simulink model "BLOC_Platform"  (R2016a)
settings: Solver=FixedStepDiscrete  StartTime=0.0  StopTime=10.0  FixedStep=hev_dt  RelTol=1e-3
undefined symbols (not defined in the file): hev_dt, pla_csat, pla_equivalent_weight, pla_f, pla_k, pla_kaero, pla_max_f_brakes, pla_wheel_radius
libraries: simulink x2
settings Model: Creator=Florent  LastModifiedBy=Florent
settings OptimizationCC: DefaultParameterBehavior=Inlined  OptimizeModelRefInitCode=on  LifeSpan=1
settings RTWCC: SystemTargetFile=ert.tlc  TemplateMakefile=ert_default_tmf  GenerateReport=on  IncludeHyperlinkInReport=on  LaunchReport=on  TargetLang=C++  GenerateTraceInfo=on  GenerateTraceReport=on  GenerateTraceReportSl=on  GenerateTraceReportSf=on  GenerateTraceReportEml=on
settings CodeAppCC: ForceParamTrailComments=on  OperatorAnnotations=on  SimulinkDataObjDesc=on  SFDataObjDesc=on  MATLABFcnDesc=on  InsertBlockDesc=on  MATLABSourceComments=on
settings ERTTargetCC: GenerateSampleERTMain=on  MultiInstanceERTCode=on  CodeInterfacePackaging=C++ class  InlinedParameterPlacement=NonHierarchical  RootIOFormat=Structure reference  ERTCustomFileTemplate=example_file_process.tlc

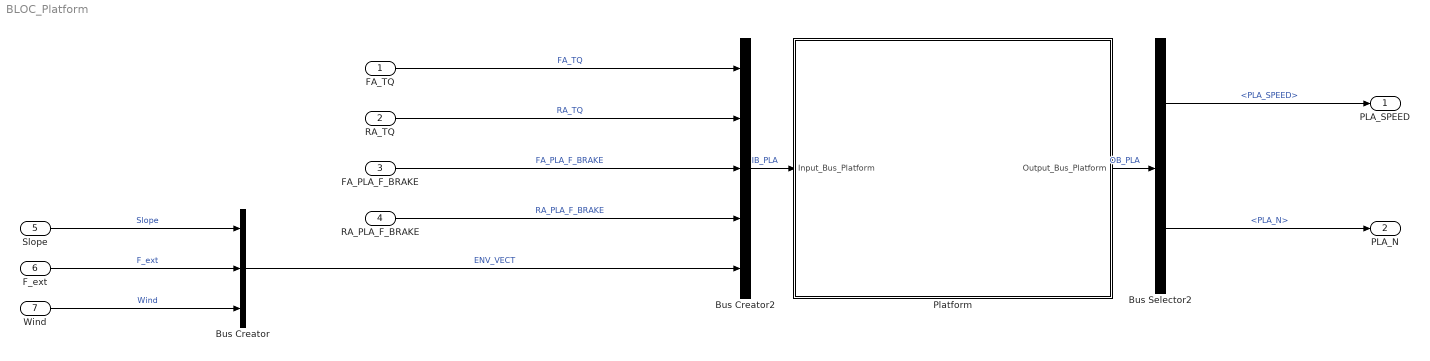
== system BLOC_Platform ==
  FA_TQ : Inport
  RA_TQ : Inport  Port=2
  FA_PLA_F_BRAKE : Inport  Port=3
  RA_PLA_F_BRAKE : Inport  Port=4
  Slope : Inport  Port=5
  F_ext : Inport  Port=6
  Wind : Inport  Port=7
  Bus Creator : BusCreator  Inputs=3
  Bus Creator2 : BusCreator  Inputs=5
  Bus Selector2 : BusSelector  OutputSignals=PLA_SPEED,PLA_N
  Platform : Subsystem  TreatAsAtomicUnit=on  SystemSampleTime=hev_dt
  PLA_SPEED : Outport
  PLA_N : Outport  Port=2
  wires:
  FA_TQ/1 -> Bus Creator2/1  "FA_TQ"
  RA_TQ/1 -> Bus Creator2/2  "RA_TQ"
  FA_PLA_F_BRAKE/1 -> Bus Creator2/3  "FA_PLA_F_BRAKE"
  RA_PLA_F_BRAKE/1 -> Bus Creator2/4  "RA_PLA_F_BRAKE"
  Bus Creator2/1 -> Platform/1(Input_Bus_Platform)  "IB_PLA"
  Platform/1(Output_Bus_Platform) -> Bus Selector2/1  "OB_PLA"
  Bus Selector2/1 -> PLA_SPEED/1  "<PLA_SPEED>"
  Bus Selector2/2 -> PLA_N/1  "<PLA_N>"
  Slope/1 -> Bus Creator/1  "Slope"
  F_ext/1 -> Bus Creator/2  "F_ext"
  Wind/1 -> Bus Creator/3  "Wind"
  Bus Creator/1 -> Bus Creator2/5  "ENV_VECT"

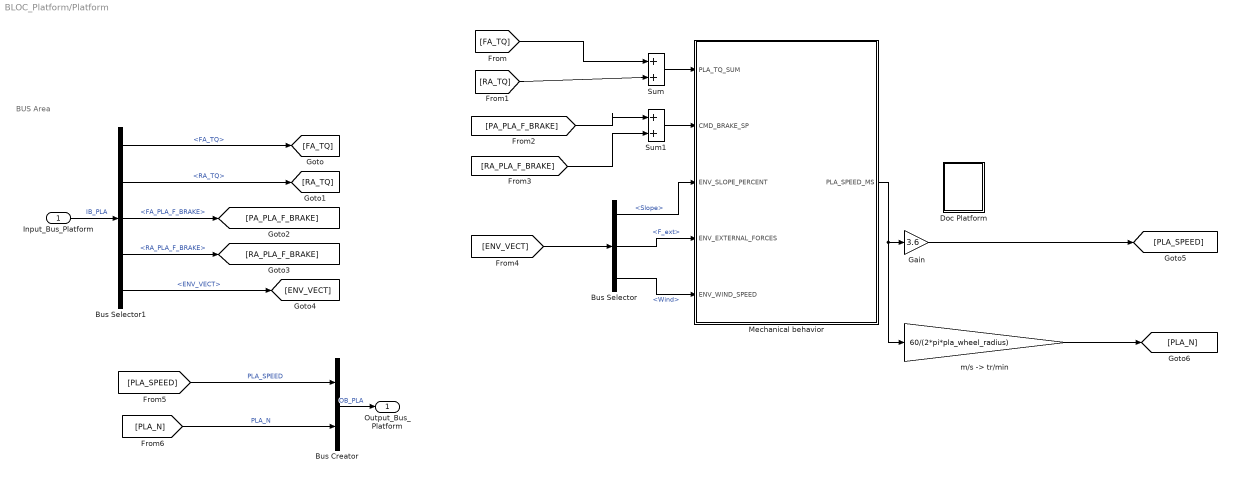
== system BLOC_Platform/Platform ==
  note: BUS Area
  Input_Bus_Platform : Inport
  Bus Creator : BusCreator  Inputs=2
  Bus Selector : BusSelector  OutputSignals=Slope,F_ext,Wind
  Bus Selector1 : BusSelector  OutputSignals=FA_TQ,RA_TQ,FA_PLA_F_BRAKE,RA_PLA_F_BRAKE,ENV_VECT
  Doc Platform : Subsystem
      settings: OpenFcn=open('Documents\Platform.pdf')
      mask Display: fprintf('DOC')
  Gain : Gain  Gain=3.6  SampleTime=hev_dt
  Mechanical behavior : Subsystem
  Sum : Sum  Inputs=+|+  SampleTime=hev_dt
  Sum1 : Sum  Inputs=+|+  SampleTime=hev_dt
  "m/s -> tr/min" : Gain  Gain=60/(2*pi*pla_wheel_radius)  SampleTime=hev_dt
  Output_Bus_Platform : Outport
  wires:
  Mechanical behavior/1(PLA_SPEED_MS) -> Gain/1, "m/s -> tr/min"/1
  [ENV_VECT] -> Bus Selector/1
  Bus Selector/1 -> Mechanical behavior/3(ENV_SLOPE_PERCENT)  "<Slope>"
  Bus Selector/2 -> Mechanical behavior/4(ENV_EXTERNAL_FORCES)  "<F_ext>"
  Bus Selector/3 -> Mechanical behavior/5(ENV_WIND_SPEED)  "<Wind>"
  Gain/1 -> [PLA_SPEED]
  "m/s -> tr/min"/1 -> [PLA_N]
  Sum/1 -> Mechanical behavior/1(PLA_TQ_SUM)
  [RA_TQ] -> Sum/2
  [FA_TQ] -> Sum/1
  Sum1/1 -> Mechanical behavior/2(CMD_BRAKE_SP)
  [RA_PLA_F_BRAKE] -> Sum1/2
  [PA_PLA_F_BRAKE] -> Sum1/1
  Input_Bus_Platform/1 -> Bus Selector1/1  "IB_PLA"
  Bus Selector1/1 -> [FA_TQ]  "<FA_TQ>"
  Bus Selector1/2 -> [RA_TQ]  "<RA_TQ>"
  Bus Selector1/3 -> [PA_PLA_F_BRAKE]  "<FA_PLA_F_BRAKE>"
  Bus Selector1/4 -> [RA_PLA_F_BRAKE]  "<RA_PLA_F_BRAKE>"
  Bus Selector1/5 -> [ENV_VECT]  "<ENV_VECT>"
  Bus Creator/1 -> Output_Bus_Platform/1  "OB_PLA"
  [PLA_SPEED] -> Bus Creator/1  "PLA_SPEED"
  [PLA_N] -> Bus Creator/2  "PLA_N"

== system BLOC_Platform/Platform/Doc Platform ==

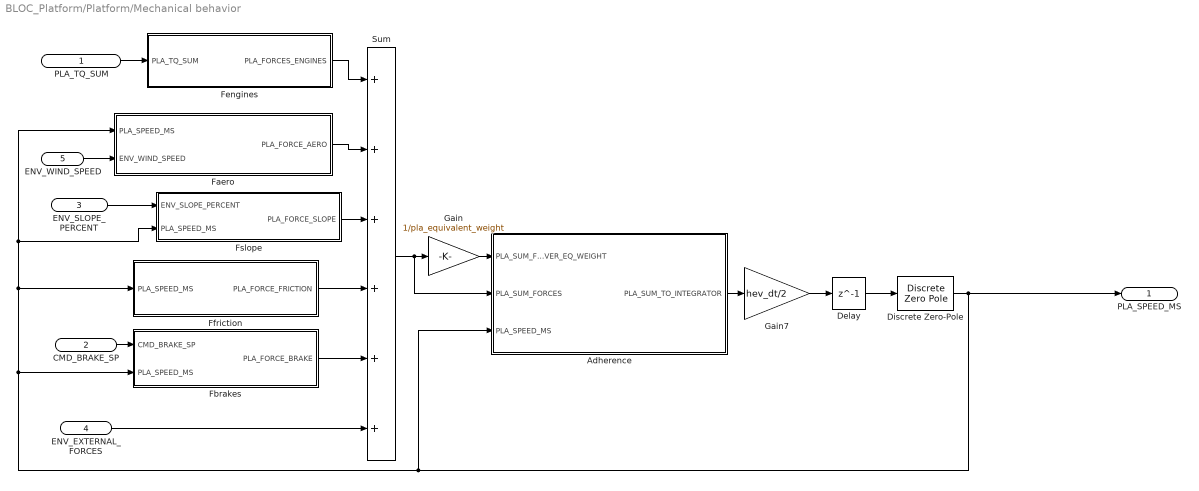
== system BLOC_Platform/Platform/Mechanical behavior ==
  PLA_TQ_SUM : Inport  Tag=tag
  CMD_BRAKE_SP : Inport  Port=2
  ENV_SLOPE_PERCENT : Inport  Port=3
  ENV_EXTERNAL_FORCES : Inport  Port=4
  ENV_WIND_SPEED : Inport  Port=5
  Adherence : Subsystem
  Delay : Delay  DelayLength=1  SampleTime=hev_dt
  Discrete Zero-Pole : DiscreteZeroPole  Zeros=[-1]  Poles=[1]  Gain=1  SampleTime=hev_dt
  Faero : Subsystem
  Fbrakes : Subsystem
  Fengines : Subsystem
  Ffriction : Subsystem
  Fslope : Subsystem
  Gain : Gain  Gain=1/pla_equivalent_weight  SampleTime=hev_dt
  Gain7 : Gain  Gain=hev_dt/2  SampleTime=hev_dt
  Sum : Sum  Inputs=++++++  SampleTime=hev_dt
  PLA_SPEED_MS : Outport
  wires:
  Gain/1 -> Adherence/1(PLA_SUM_FORCES_OVER_EQ_WEIGHT)
  Ffriction/1(PLA_FORCE_FRICTION) -> Sum/4
  Sum/1 -> Gain/1, Adherence/2(PLA_SUM_FORCES)
  Discrete Zero-Pole/1 -> Adherence/3(PLA_SPEED_MS), Fbrakes/2(PLA_SPEED_MS), Ffriction/1(PLA_SPEED_MS), Faero/1(PLA_SPEED_MS), Fslope/2(PLA_SPEED_MS), PLA_SPEED_MS/1
  ENV_SLOPE_PERCENT/1 -> Fslope/1(ENV_SLOPE_PERCENT)
  ENV_WIND_SPEED/1 -> Faero/2(ENV_WIND_SPEED)
  PLA_TQ_SUM/1 -> Fengines/1(PLA_TQ_SUM)
  Fengines/1(PLA_FORCES_ENGINES) -> Sum/1
  Faero/1(PLA_FORCE_AERO) -> Sum/2
  Fslope/1(PLA_FORCE_SLOPE) -> Sum/3
  ENV_EXTERNAL_FORCES/1 -> Sum/6
  CMD_BRAKE_SP/1 -> Fbrakes/1(CMD_BRAKE_SP)
  Fbrakes/1(PLA_FORCE_BRAKE) -> Sum/5
  Adherence/1(PLA_SUM_TO_INTEGRATOR) -> Gain7/1
  Gain7/1 -> Delay/1
  Delay/1 -> Discrete Zero-Pole/1

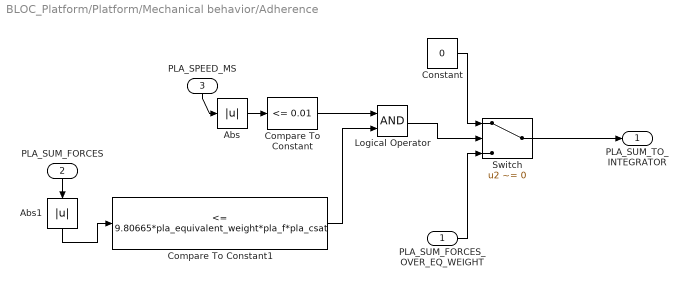
== system BLOC_Platform/Platform/Mechanical behavior/Adherence ==
  PLA_SUM_FORCES_OVER_EQ_WEIGHT : Inport
  PLA_SUM_FORCES : Inport  Port=2
  PLA_SPEED_MS : Inport  Port=3
  Abs : Abs  SampleTime=hev_dt
  Abs1 : Abs  SampleTime=hev_dt
  Compare To Constant : simulink/Logic and Bit Operations/Compare To Constant  relop=<=  const=0.01  OutDataTypeStr=uint8
  Compare To Constant1 : simulink/Logic and Bit Operations/Compare To Constant  relop=<=  const=9.80665*pla_equivalent_weight*pla_f*pla_csat  OutDataTypeStr=uint8
  Constant : Constant  Value=0
  Logical Operator : Logic  AllPortsSameDT=off  OutDataTypeStr=boolean  SampleTime=hev_dt
  Switch : Switch  Criteria=u2 ~= 0  SampleTime=hev_dt
  PLA_SUM_TO_INTEGRATOR : Outport
  wires:
  PLA_SUM_FORCES_OVER_EQ_WEIGHT/1 -> Switch/3
  Switch/1 -> PLA_SUM_TO_INTEGRATOR/1
  PLA_SPEED_MS/1 -> Abs/1
  PLA_SUM_FORCES/1 -> Abs1/1
  Abs1/1 -> Compare To Constant1/1
  Abs/1 -> Compare To Constant/1
  Constant/1 -> Switch/1
  Compare To Constant1/1 -> Logical Operator/2
  Logical Operator/1 -> Switch/2
  Compare To Constant/1 -> Logical Operator/1

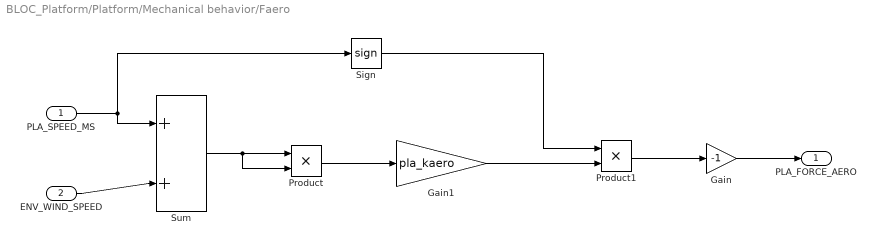
== system BLOC_Platform/Platform/Mechanical behavior/Faero ==
  PLA_SPEED_MS : Inport
  ENV_WIND_SPEED : Inport  Port=2
  Gain : Gain  Gain=-1  SampleTime=hev_dt
  Gain1 : Gain  Gain=pla_kaero  SampleTime=hev_dt
  Product : Product  SampleTime=hev_dt
  Product1 : Product  SampleTime=hev_dt
  Sign : Signum  SampleTime=hev_dt
  Sum : Sum  Inputs=+|+  SampleTime=hev_dt
  PLA_FORCE_AERO : Outport
  wires:
  PLA_SPEED_MS/1 -> Sign/1, Sum/1
  ENV_WIND_SPEED/1 -> Sum/2
  Sum/1 -> Product/2, Product/1
  Product/1 -> Gain1/1
  Gain1/1 -> Product1/2
  Product1/1 -> Gain/1
  Sign/1 -> Product1/1
  Gain/1 -> PLA_FORCE_AERO/1

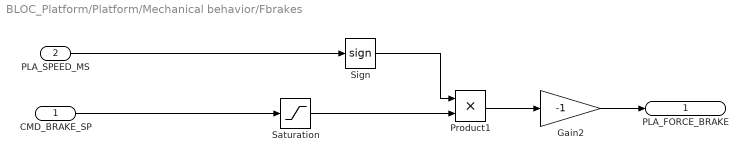
== system BLOC_Platform/Platform/Mechanical behavior/Fbrakes ==
  CMD_BRAKE_SP : Inport
  PLA_SPEED_MS : Inport  Port=2
  Gain2 : Gain  Gain=-1  SampleTime=hev_dt
  Product1 : Product  SampleTime=hev_dt
  Saturation : Saturate  UpperLimit=pla_max_f_brakes  LowerLimit=0
  Sign : Signum  SampleTime=hev_dt
  PLA_FORCE_BRAKE : Outport
  wires:
  CMD_BRAKE_SP/1 -> Saturation/1
  PLA_SPEED_MS/1 -> Sign/1
  Sign/1 -> Product1/1
  Product1/1 -> Gain2/1
  Gain2/1 -> PLA_FORCE_BRAKE/1
  Saturation/1 -> Product1/2

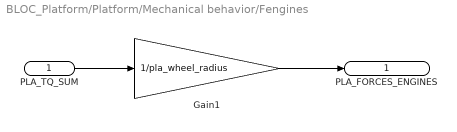
== system BLOC_Platform/Platform/Mechanical behavior/Fengines ==
  PLA_TQ_SUM : Inport
  Gain1 : Gain  Gain=1/pla_wheel_radius  SampleTime=hev_dt
  PLA_FORCES_ENGINES : Outport
  wires:
  PLA_TQ_SUM/1 -> Gain1/1
  Gain1/1 -> PLA_FORCES_ENGINES/1

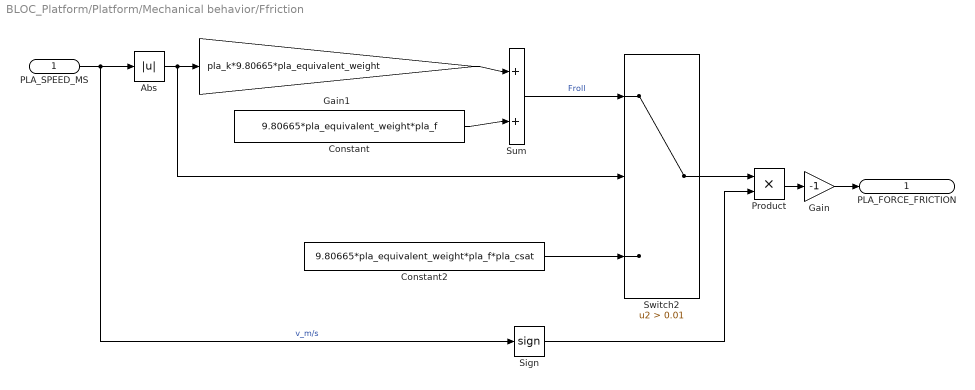
== system BLOC_Platform/Platform/Mechanical behavior/Ffriction ==
  PLA_SPEED_MS : Inport
  Abs : Abs  SampleTime=hev_dt
  Constant : Constant  Value=9.80665*pla_equivalent_weight*pla_f
  Constant2 : Constant  Value=9.80665*pla_equivalent_weight*pla_f*pla_csat
  Gain : Gain  Gain=-1  SampleTime=hev_dt
  Gain1 : Gain  Gain=pla_k*9.80665*pla_equivalent_weight  SampleTime=hev_dt
  Product : Product  SampleTime=hev_dt
  Sign : Signum  SampleTime=hev_dt
  Sum : Sum  Inputs=+|+  SampleTime=hev_dt
  Switch2 : Switch  Criteria=u2 > Threshold  Threshold=0.01  SampleTime=hev_dt
  PLA_FORCE_FRICTION : Outport
  wires:
  PLA_SPEED_MS/1 -> Abs/1, Sign/1  "v_m/s"
  Gain1/1 -> Sum/1
  Constant/1 -> Sum/2
  Abs/1 -> Gain1/1, Switch2/2
  Switch2/1 -> Product/1
  Product/1 -> Gain/1
  Sign/1 -> Product/2
  Gain/1 -> PLA_FORCE_FRICTION/1
  Sum/1 -> Switch2/1  "Froll"
  Constant2/1 -> Switch2/3

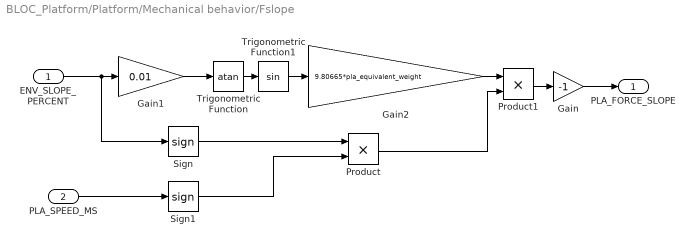
== system BLOC_Platform/Platform/Mechanical behavior/Fslope ==
  ENV_SLOPE_PERCENT : Inport
  PLA_SPEED_MS : Inport  Port=2
  Gain : Gain  Gain=-1  SampleTime=hev_dt
  Gain1 : Gain  Gain=0.01  SampleTime=hev_dt
  Gain2 : Gain  Gain=9.80665*pla_equivalent_weight  SampleTime=hev_dt
  Product : Product  SampleTime=hev_dt
  Product1 : Product  SampleTime=hev_dt
  Sign : Signum  SampleTime=hev_dt
  Sign1 : Signum  SampleTime=hev_dt
  Trigonometric Function : Trigonometry  Operator=atan  SampleTime=hev_dt
  Trigonometric Function1 : Trigonometry  SampleTime=hev_dt
  PLA_FORCE_SLOPE : Outport
  wires:
  ENV_SLOPE_PERCENT/1 -> Sign/1, Gain1/1
  Gain1/1 -> Trigonometric Function/1
  Trigonometric Function/1 -> Trigonometric Function1/1
  Trigonometric Function1/1 -> Gain2/1
  Gain/1 -> PLA_FORCE_SLOPE/1
  PLA_SPEED_MS/1 -> Sign1/1
  Sign/1 -> Product/1
  Sign1/1 -> Product/2
  Gain2/1 -> Product1/1
  Product/1 -> Product1/2
  Product1/1 -> Gain/1
